simulink model "Assemblaggio"  (R2019a)
settings: Solver=VariableStepAuto  StartTime=0.0  StopTime=10.0  RelTol=1e-3
settings Model: Creator=anton  LastModifiedBy=anton

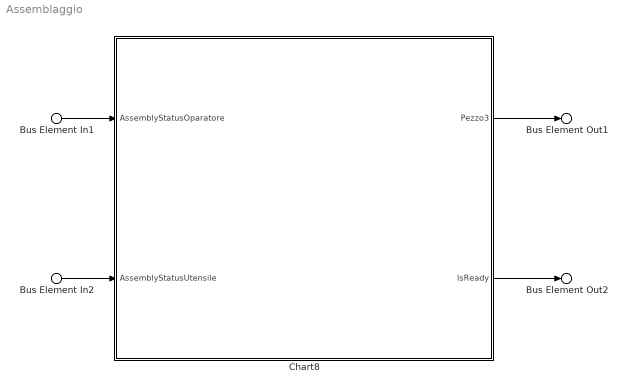
== system Assemblaggio ==
  Bus Element In1 : Inport  PortName=AssemblyStatusOperatore
  Bus Element In2 : Inport  Port=2  PortName=AssemblyStatusUtensile
  Chart8 : Stateflow chart  BlockKeywords=__PRM__SERIALIZED__DATA__:Stateflow Chart,Stateflow Diagram  TreatAsAtomicUnit=on
  Bus Element Out1 : Outport  PortName=Pezzo3
  Bus Element Out2 : Outport  Port=2  PortName=IsReady
  wires:
  Bus Element In1/1 -> Chart8/1(AssemblyStatusOparatore)
  Chart8/1(Pezzo3) -> Bus Element Out1/1
  Chart8/2(IsReady) -> Bus Element Out2/1
  Bus Element In2/1 -> Chart8/2(AssemblyStatusUtensile)

== stateflow chart Assemblaggio/Chart8 ==
  state Montage
    if AssemblyStatusOparatore == 1 || AssemblyStatusUtensile == 1
    IsReady = 1;
    Pezzo3 = 1;
    end
  (default) -> Montage
  data: Pezzo3 output; IsReady output; AssemblyStatusOparatore input; AssemblyStatusUtensile input
